simulink model "Respueste_en_tiempo"  (Simulink 10.2)
settings: Solver=ode45  StartTime=0.0  StopTime=3  RelTol=1e-6  EnableMultiTasking=on
values from neighbouring files (symbols this model uses):
  Ck = 14.27    [TEORICO_Respuesta_en_frecuencia.m]
  Cp = 0.84    [TEORICO_Respuesta_en_frecuencia.m]
  Kd = 0    [TEORICO_Respuesta_en_frecuencia.m]
  Ki = 1    [TEORICO_Respuesta_en_frecuencia.m]
  Kp = 0.15    [TEORICO_Respuesta_en_frecuencia.m]
libraries: simulink_need_slupdate x1
settings Model: Creator=Rober  LastModifiedBy=diego
settings DataIOCC: LimitDataPoints=on
settings OptimizationCC: ExpressionDepthLimit=2147483647  InitFltsAndDblsToZero=on
settings DebuggingCC: SaveWithParameterizedLinksMsg=none  SignalResolutionControl=TryResolveAllWithWarning  SolverPrmCheckMsg=warning  MultiTaskDSMMsg=warning  MultiTaskCondExecSysMsg=none  StateNameClashWarn=warning
settings GRTTargetCC: TargetFcnLib=ansi_tfl_tmw.mat
settings ConfigComp: CovSFcnEnable=off

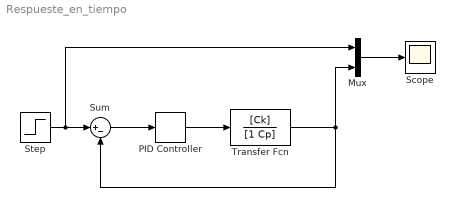
== system Respueste_en_tiempo ==
  Mux : Mux  Inputs=2
  PID Controller : simulink_need_slupdate/PID Controller  P=Kp  I=Ki  D=Kd
  Scope : Scope
  Step : Step  Time=0  SampleTime=0
  Sum : Sum  Inputs=|+-
  Transfer Fcn : TransferFcn  Numerator=[Ck]  Denominator=[1 Cp]
  wires:
  Transfer Fcn/1 -> Mux/2, Sum/2
  Step/1 -> Sum/1, Mux/1
  Mux/1 -> Scope/1
  PID Controller/1 -> Transfer Fcn/1
  Sum/1 -> PID Controller/1
